simulink model "airframeDynamics"  (R2015a)
settings: Solver=ode45  StartTime=0.0  StopTime=20.0  FixedStep=.001  MaxStep=.01  RelTol=1e-3
values from neighbouring files (symbols this model uses):
  h_body_int_init : value not decoded    [plantDynamicsDictionary.sldd]
  I_body : value not decoded    [plantDynamicsDictionary.sldd]
  I_body_inverse : value not decoded    [plantDynamicsDictionary.sldd]
  MASS = 2.0    [plantDynamicsDictionary.sldd]
  q_body_NED_init : value not decoded    [plantDynamicsDictionary.sldd]
  w_body_init : value not decoded    [plantDynamicsDictionary.sldd]
  x_init_ECEF : value not decoded    [plantDynamicsDictionary.sldd]
libraries: QuaternionLibrary x3, VectorLibrary x1
settings Model: DataDictionary=plantDynamicsDictionary.sldd  Creator=Cam  LastModifiedBy=Cam

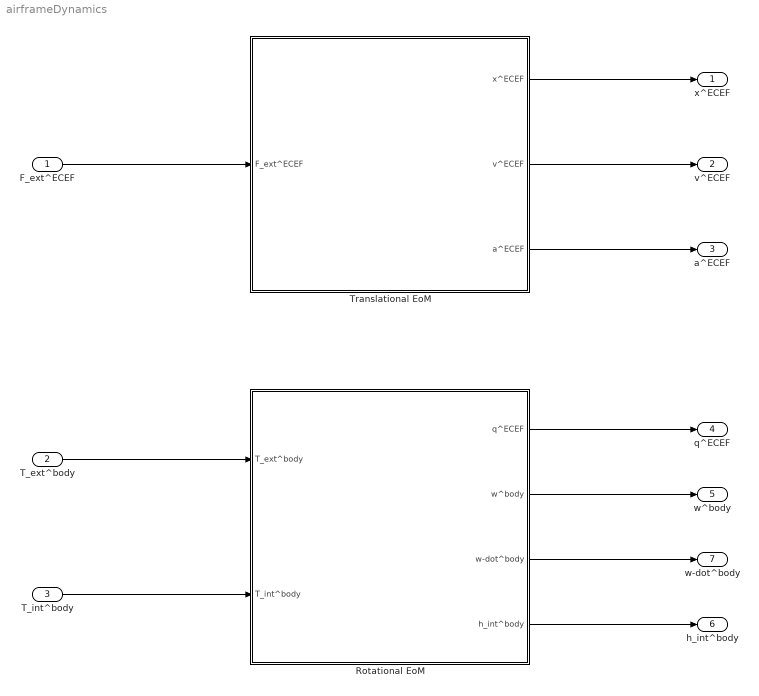
== system airframeDynamics ==
  F_ext^ECEF : Inport
  T_ext^body : Inport  Port=2
  T_int^body : Inport  Port=3
  Rotational EoM : Subsystem
  Translational EoM : Subsystem
  x^ECEF : Outport
  v^ECEF : Outport  Port=2
  a^ECEF : Outport  Port=3
  q^ECEF : Outport  Port=4
  w^body : Outport  Port=5
  h_int^body : Outport  Port=6
  w-dot^body : Outport  Port=7
  wires:
  F_ext^ECEF/1 -> Translational EoM/1(F_ext^ECEF)
  Translational EoM/1(x^ECEF) -> x^ECEF/1
  Translational EoM/2(v^ECEF) -> v^ECEF/1
  Translational EoM/3(a^ECEF) -> a^ECEF/1
  T_ext^body/1 -> Rotational EoM/1(T_ext^body)
  T_int^body/1 -> Rotational EoM/2(T_int^body)
  Rotational EoM/1(q^ECEF) -> q^ECEF/1
  Rotational EoM/2(w^body) -> w^body/1
  Rotational EoM/4(h_int^body) -> h_int^body/1
  Rotational EoM/3(w-dot^body) -> w-dot^body/1

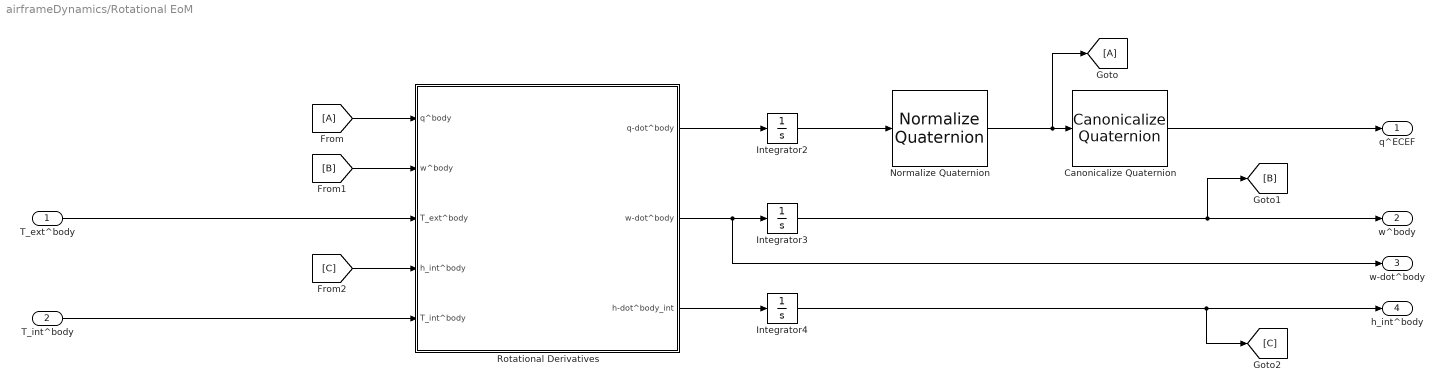
== system airframeDynamics/Rotational EoM ==
  T_ext^body : Inport
  T_int^body : Inport  Port=2
  Canonicalize Quaternion : QuaternionLibrary/Canonicalize Quaternion
  Integrator2 : Integrator  InitialCondition=q_body_NED_init
  Integrator3 : Integrator  InitialCondition=w_body_init
  Integrator4 : Integrator  InitialCondition=h_body_int_init
  Normalize Quaternion : QuaternionLibrary/Normalize Quaternion
  Rotational Derivatives : Subsystem
  q^ECEF : Outport
  w^body : Outport  Port=2
  w-dot^body : Outport  Port=3
  h_int^body : Outport  Port=4
  wires:
  T_ext^body/1 -> Rotational Derivatives/3(T_ext^body)
  T_int^body/1 -> Rotational Derivatives/5(T_int^body)
  Canonicalize Quaternion/1 -> q^ECEF/1
  Rotational Derivatives/3(h-dot^body_int) -> Integrator4/1
  [B] -> Rotational Derivatives/2(w^body)
  [C] -> Rotational Derivatives/4(h_int^body)
  [A] -> Rotational Derivatives/1(q^body)
  Rotational Derivatives/2(w-dot^body) -> w-dot^body/1, Integrator3/1
  Integrator3/1 -> w^body/1, [B]
  Integrator4/1 -> h_int^body/1, [C]
  Integrator2/1 -> Normalize Quaternion/1
  Normalize Quaternion/1 -> [A], Canonicalize Quaternion/1
  Rotational Derivatives/1(q-dot^body) -> Integrator2/1

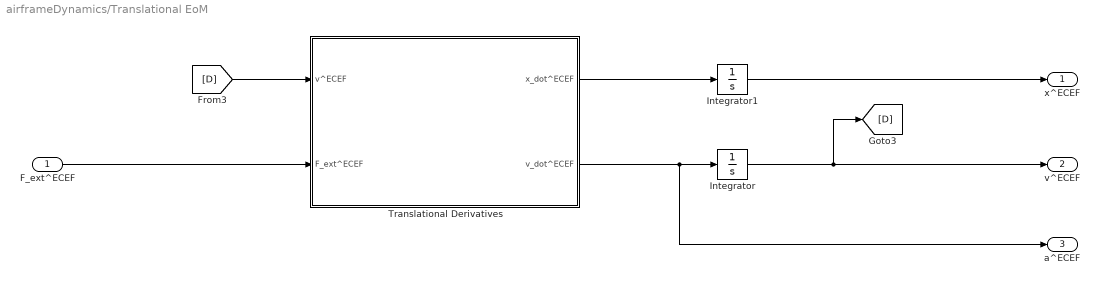
== system airframeDynamics/Translational EoM ==
  F_ext^ECEF : Inport
  Integrator : Integrator  InitialCondition=[0 0 0]
  Integrator1 : Integrator  InitialCondition=x_init_ECEF
  Translational Derivatives : Subsystem
  x^ECEF : Outport
  v^ECEF : Outport  Port=2
  a^ECEF : Outport  Port=3
  wires:
  [D] -> Translational Derivatives/1(v^ECEF)
  Integrator1/1 -> x^ECEF/1
  Translational Derivatives/2(v_dot^ECEF) -> a^ECEF/1, Integrator/1
  Translational Derivatives/1(x_dot^ECEF) -> Integrator1/1
  Integrator/1 -> v^ECEF/1, [D]
  F_ext^ECEF/1 -> Translational Derivatives/2(F_ext^ECEF)

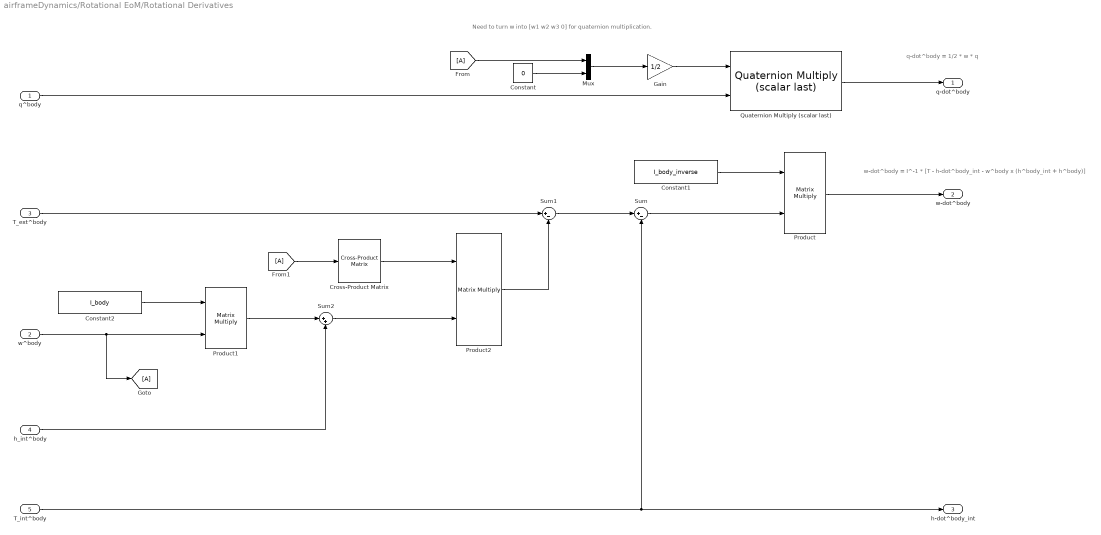
== system airframeDynamics/Rotational EoM/Rotational Derivatives ==
  note: w-dot^body = I^-1 * [T - h-dot^body_int - w^body x (h^body_int + h^body)]
  note: q-dot^body = 1/2 * w * q
  note: Need to turn w into [w1 w2 w3 0] for quaternion multiplication.
  q^body : Inport
  w^body : Inport  Port=2
  T_ext^body : Inport  Port=3  PortDimensions=3
  h_int^body : Inport  Port=4
  T_int^body : Inport  Port=5  PortDimensions=3
  Constant : Constant  Value=0
  Constant1 : Constant  Value=I_body_inverse
  Constant2 : Constant  Value=I_body
  Cross-Product Matrix : VectorLibrary/Cross-Product Matrix
  Gain : Gain  Gain=1/2
  Mux : Mux  Inputs=2
  Product : Product  Multiplication=Matrix(*)
  Product1 : Product  Multiplication=Matrix(*)
  Product2 : Product  Multiplication=Matrix(*)
  Quaternion Multiply (scalar last) : QuaternionLibrary/Quaternion Math/Quaternion Multiply (scalar last)
  Sum : Sum  Inputs=|+-
  Sum1 : Sum  Inputs=|+-
  Sum2 : Sum  Inputs=|++
  q-dot^body : Outport
  w-dot^body : Outport  Port=2
  h-dot^body_int : Outport  Port=3
  wires:
  Gain/1 -> Quaternion Multiply (scalar last)/1
  q^body/1 -> Quaternion Multiply (scalar last)/2
  w^body/1 -> Product1/2, [A]
  Mux/1 -> Gain/1
  Constant/1 -> Mux/2
  [A] -> Mux/1
  Sum/1 -> Product/2
  Constant1/1 -> Product/1
  Product/1 -> w-dot^body/1
  Sum1/1 -> Sum/1
  T_ext^body/1 -> Sum1/1
  Product1/1 -> Sum2/1
  h_int^body/1 -> Sum2/2
  Constant2/1 -> Product1/1
  Sum2/1 -> Product2/2
  Cross-Product Matrix/1 -> Product2/1
  [A] -> Cross-Product Matrix/1
  Product2/1 -> Sum1/2
  T_int^body/1 -> Sum/2, h-dot^body_int/1
  Quaternion Multiply (scalar last)/1 -> q-dot^body/1

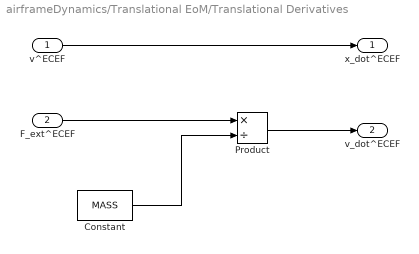
== system airframeDynamics/Translational EoM/Translational Derivatives ==
  v^ECEF : Inport
  F_ext^ECEF : Inport  Port=2  PortDimensions=3
  Constant : Constant  Value=MASS
  Product : Product  Inputs=*/
  x_dot^ECEF : Outport
  v_dot^ECEF : Outport  Port=2
  wires:
  Constant/1 -> Product/2
  F_ext^ECEF/1 -> Product/1
  v^ECEF/1 -> x_dot^ECEF/1
  Product/1 -> v_dot^ECEF/1
